simulink model "NHCtrl"  (R2017b)
settings: Solver=ode4  StartTime=0.0  StopTime=20  FixedStep=sim_step  RelTol=1e-3  EnableMultiTasking=on
undefined symbols (not defined in the file): g, J, kd, kd_z, KDP, KDR, KDY, ki, kp, KPP, KPR, m, max_pos_err_norm, max_tilt
settings Model: Creator=Burak  LastModifiedBy=buyue
settings DataIOCC: LimitDataPoints=on  SaveFormat=Array
settings OptimizationCC: LifeSpan=inf
settings DebuggingCC: UnderspecifiedInitializationDetection=Classic  MergeDetectMultiDrivingBlocksExec=none  SolverPrmCheckMsg=warning  StateNameClashWarn=warning  SFUnexpectedBacktrackingDiag=warning  SFNoUnconditionalDefaultTransitionDiag=warning  SFExecutionAtInitializationDiag=none
settings HardwareCC: ProdBitPerPointer=32  ProdBitPerSizeT=32  ProdBitPerPtrDiffT=32  ProdLargestAtomicFloat=None  ProdIntDivRoundTo=Undefined  ProdEndianess=Unspecified  ProdWordSize=32  ProdHWDeviceType=32-bit Generic
settings ModelReferenceCC: PropagateSignalLabelsOutOfModel=off
settings CodeAppCC: StateflowObjectComments=on
settings GRTTargetCC: TargetLangStandard=C89/C90 (ANSI)  GeneratePreprocessorConditionals=Disable all
settings ConfigComp: CovMetricSettings=dw  CovHtmlReporting=on  CovSaveCumulativeToWorkspaceVar=on  CovSaveSingleToWorkspaceVar=on  CovExternalEMLEnable=off

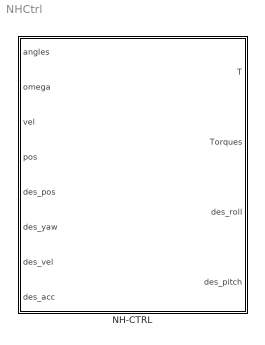
== system NHCtrl ==
  NH-CTRL : Subsystem  Description=|
      | % Near-Hovering Controller.
      | % Code part of Lecture IAR @IST-Uni Stuttgart
      | % Author: Burak Yueksel
      | % Author: Antonio Franchi

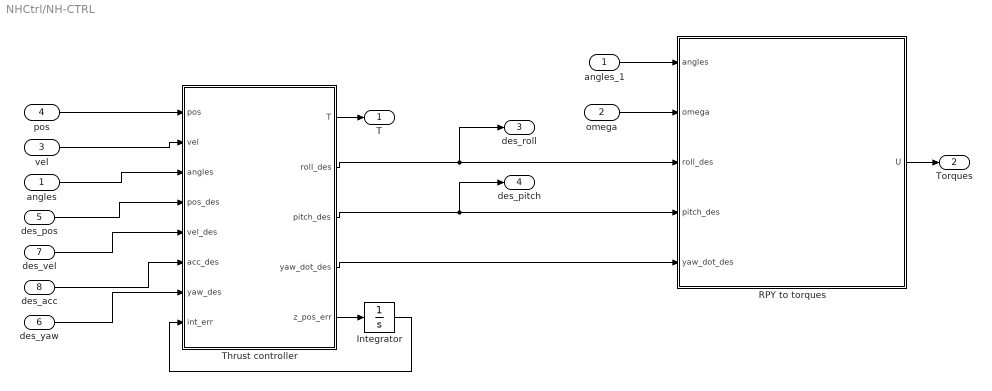
== system NHCtrl/NH-CTRL ==
  angles : Inport
  omega : Inport  Port=2
  vel : Inport  Port=3
  pos : Inport  Port=4
  des_pos : Inport  Port=5
  des_yaw : Inport  Port=6
  des_vel : Inport  Port=7
  des_acc : Inport  Port=8
  Integrator : Integrator
  RPY to torques : MATLAB Function  Description=|  TreatAsAtomicUnit=on
      | % Rotational part of the Near-Hovering Controller.
      | % Code part of Lecture IAR @IST-Uni Stuttgart
      | % Author: Burak Yueksel
      | % Author: Antonio Franchi
  Thrust controller : MATLAB Function  Description=|  TreatAsAtomicUnit=on
      | % Translational part of the Near-Hovering Controller.
      | % Code part of Lecture IAR @IST-Uni Stuttgart
      | % Author: Burak Yueksel
      | % Author: Antonio Franchi
  angles_1 : InportShadow
  T : Outport
  Torques : Outport  Port=2
  des_roll : Outport  Port=3
  des_pitch : Outport  Port=4
  wires:
  Integrator/1 -> Thrust controller/8(int_err)
  omega/1 -> RPY to torques/2(omega)
  vel/1 -> Thrust controller/2(vel)
  Thrust controller/3(pitch_des) -> des_pitch/1, RPY to torques/4(pitch_des)
  Thrust controller/4(yaw_dot_des) -> RPY to torques/5(yaw_dot_des)
  angles_1/1 -> RPY to torques/1(angles)
  des_acc/1 -> Thrust controller/6(acc_des)
  des_pos/1 -> Thrust controller/4(pos_des)
  des_yaw/1 -> Thrust controller/7(yaw_des)
  pos/1 -> Thrust controller/1(pos)
  Thrust controller/2(roll_des) -> des_roll/1, RPY to torques/3(roll_des)
  angles/1 -> Thrust controller/3(angles)
  Thrust controller/5(z_pos_err) -> Integrator/1
  des_vel/1 -> Thrust controller/5(vel_des)
  RPY to torques/1(U) -> Torques/1
  Thrust controller/1(T) -> T/1

== matlab function NHCtrl/NH-CTRL/RPY to torques ==
  data: angles input; U output; omega input; roll_des input; pitch_des input; yaw_dot_des input; J parameter; KDR parameter; KPR parameter; KDP parameter; KPP parameter; KDY parameter
function U  = fcn(angles, omega, roll_des, pitch_des, yaw_dot_des, J, KDR, KPR, KDP, KPP, KDY)
% Rotational part of the Near-Hovering Controller.
% Code part of Lecture IAR @IST-Uni Stuttgart
% Author: Burak Yueksel
% Author: Antonio Franchi
%
% Initiate the torques
U=[0;0;0];
% Get Euler angles
r = angles(1);
p = angles(2);
y=angles(3);
% Transformation matrix from body frame velocities to the Euler rates
T = [1      tan(p)*sin(r) tan(p)*cos(r);
    0       cos(r)  -sin(r);
    0       sin(r)/cos(p)   cos(r)/cos(p)];
% From body frame velocities to Euler rates
dot_ang = T*omega;
% Separate euler rates
dot_r = dot_ang(1);
dot_p = dot_ang(2);
dot_y = dot_ang(3);
% skew-symmetric form of body frame velocities
% hat operation: R3->so3 (inverse of vee)
Sw = [0 -omega(3) omega(2);                         
      omega(3) 0 -omega(1);
     -omega(2) omega(1) 0];
% Compute the torques
% Notice that T^{-1} is analytically defined. You can use it instead of
% numerical inverse
U=Sw*J*omega + J*inv(T)*([ KDR * (0 - dot_r) + KPR * (roll_des - r); KDP * (0 - dot_p) + KPP * (pitch_des - p) ; KDY * (yaw_dot_des - dot_y) ]);

== matlab function NHCtrl/NH-CTRL/Thrust controller ==
  data: pos input; vel input; angles input; pos_des input; g parameter; m parameter; T output; roll_des output; pitch_des output; vel_des input; acc_des input; yaw_des input; yaw_dot_des output; kd parameter; kp parameter; ki parameter; max_tilt parameter; kd_z parameter; max_pos_err_norm parameter; int_err input; z_pos_err output
function [T, roll_des, pitch_des, yaw_dot_des,z_pos_err] = fcn(pos, vel, angles, pos_des, g, m, vel_des, acc_des,yaw_des, kd, kp, ki, max_tilt, kd_z, max_pos_err_norm,int_err)
% Translational part of the Near-Hovering Controller.
% Code part of Lecture IAR @IST-Uni Stuttgart
% Author: Burak Yueksel
% Author: Antonio Franchi
%
% get euler angles
r = angles(1);
p = angles(2);
y = angles(3);
% get position error
pos_err = pos_des-pos;
% init thrust forces
T=zeros(3,1);
%soft saturation on position error
sat_norm = (2*max_pos_err_norm/pi) * atan( pi* norm(pos_err) / (2*max_pos_err_norm) );
if norm(pos_err) > 0.0001
    pos_err = pos_err/norm(pos_err) * sat_norm;
end
% compute thrust forces. Notice that for altitude an integrator term is
% added
T=[0;0;m/(cos(r)*cos(p))*(-g+ acc_des(3) + kd_z*(vel_des(3) -vel(3)) + kp*(pos_err(3)) +ki*int_err )];
% desired x-y acc are set to zero. Compute x y accelerations from position
% and velocity errors
ddpx=kd*(vel_des(1) -vel(1)) + kp*(pos_err(1));
ddpy=kd*(vel_des(2) -vel(2)) + kp*(pos_err(2));
% maximum roll and pitch angles
max_roll=sin(max_tilt);
max_pitch=sin(max_tilt);
% control roll and pitch: \sin(\phi^d) and \sin(\theta^d)
ctrl_roll=m/T(3)*( -sin(y)*ddpx+cos(y)*ddpy);
ctrl_pitch= m/(T(3)*cos(r))*( cos(y)*ddpx+sin(y)*ddpy);
%soft saturation on control roll and pitch values
ctrl_roll = (2*max_roll/pi) * atan( pi* ctrl_roll / (2*max_roll) );
ctrl_pitch = (2*max_pitch/pi) * atan( pi* ctrl_pitch / (2*max_pitch) );
% get the roll and pitch angles
roll_des = -asin(ctrl_roll);
pitch_des = asin(ctrl_pitch);
% altitude error to be integrated over time
z_pos_err = pos_err(3);
% desired yaw rate computed from yaw error
yaw_dot_des = kp*atan2(sin(yaw_des-y),cos(yaw_des-y));
